simulink model "Zad2"  (R2020b)
settings: Solver=FixedStepAuto  StartTime=0.0  StopTime=200  FixedStep=0.1  RelTol=1e-3
undefined symbols (not defined in the file): kr, Tp
settings Model: Creator=Maciek  LastModifiedBy=Maciek

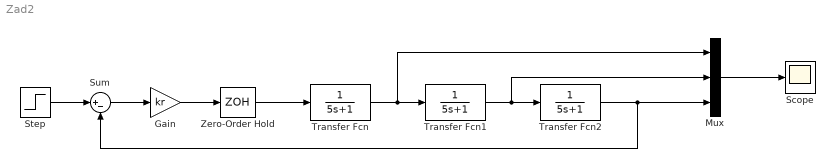
== system Zad2 ==
  Gain : Gain  Gain=kr
  Mux : Mux  Inputs=3
  Scope : Scope
  Step : Step  SampleTime=0
  Sum : Sum  Inputs=|+-
  Transfer Fcn : TransferFcn  Denominator=[5 1]
  Transfer Fcn1 : TransferFcn  Denominator=[5 1]
  Transfer Fcn2 : TransferFcn  Denominator=[5 1]
  Zero-Order Hold : ZeroOrderHold  SampleTime=Tp
  wires:
  Step/1 -> Sum/1
  Mux/1 -> Scope/1
  Transfer Fcn2/1 -> Sum/2, Mux/3
  Transfer Fcn/1 -> Mux/1, Transfer Fcn1/1
  Zero-Order Hold/1 -> Transfer Fcn/1
  Gain/1 -> Zero-Order Hold/1
  Sum/1 -> Gain/1
  Transfer Fcn1/1 -> Mux/2, Transfer Fcn2/1
